simulink model "TST_Rail_CtlLoopParaMeUn"  (R2016b)
settings: Solver=FixedStepDiscrete  StartTime=0.0  StopTime=simTime  FixedStep=sampleTime  RelTol=1e-3
values from neighbouring files (symbols this model uses):
  testCase = 1    [initTST_Rail_CtlLoopParaMeUn_001.m]
libraries: simulink x11, UnitTest_Lib x9
settings Model: Creator=zhengjinyan  LastModifiedBy=zhengjinyan
settings DebuggingCC: SignalRangeChecking=error

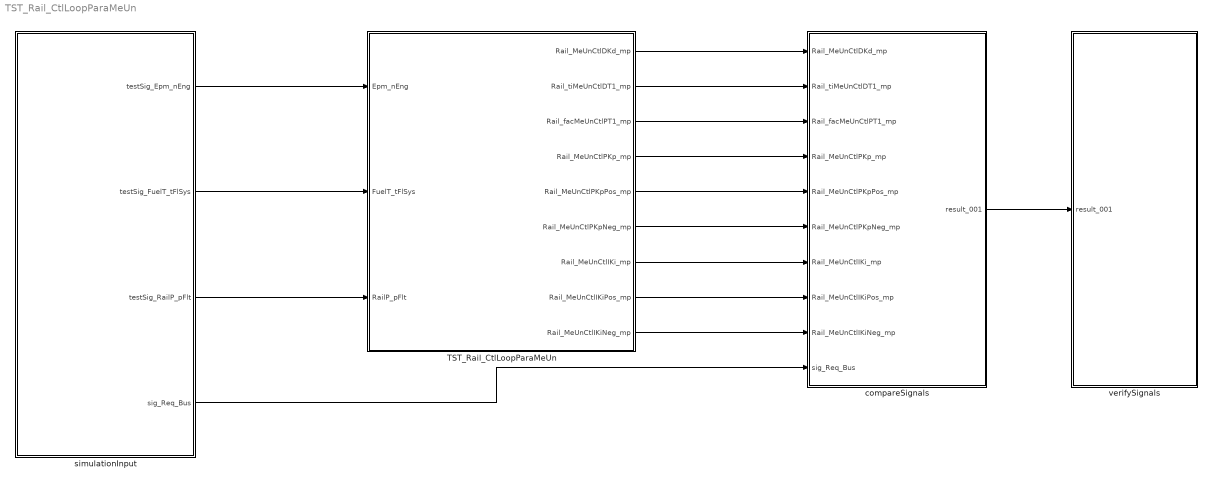
== system TST_Rail_CtlLoopParaMeUn ==
  TST_Rail_CtlLoopParaMeUn : Subsystem
  compareSignals : Subsystem
  simulationInput : Subsystem
  verifySignals : Subsystem
  wires:
  simulationInput/1(testSig_Epm_nEng) -> TST_Rail_CtlLoopParaMeUn/1(Epm_nEng)
  simulationInput/2(testSig_FuelT_tFlSys) -> TST_Rail_CtlLoopParaMeUn/2(FuelT_tFlSys)
  simulationInput/3(testSig_RailP_pFlt) -> TST_Rail_CtlLoopParaMeUn/3(RailP_pFlt)
  TST_Rail_CtlLoopParaMeUn/1(Rail_MeUnCtlDKd_mp) -> compareSignals/1(Rail_MeUnCtlDKd_mp)
  TST_Rail_CtlLoopParaMeUn/2(Rail_tiMeUnCtlDT1_mp) -> compareSignals/2(Rail_tiMeUnCtlDT1_mp)
  TST_Rail_CtlLoopParaMeUn/3(Rail_facMeUnCtlPT1_mp) -> compareSignals/3(Rail_facMeUnCtlPT1_mp)
  TST_Rail_CtlLoopParaMeUn/4(Rail_MeUnCtlPKp_mp) -> compareSignals/4(Rail_MeUnCtlPKp_mp)
  TST_Rail_CtlLoopParaMeUn/5(Rail_MeUnCtlPKpPos_mp) -> compareSignals/5(Rail_MeUnCtlPKpPos_mp)
  TST_Rail_CtlLoopParaMeUn/6(Rail_MeUnCtlPKpNeg_mp) -> compareSignals/6(Rail_MeUnCtlPKpNeg_mp)
  TST_Rail_CtlLoopParaMeUn/7(Rail_MeUnCtlIKi_mp) -> compareSignals/7(Rail_MeUnCtlIKi_mp)
  TST_Rail_CtlLoopParaMeUn/8(Rail_MeUnCtlIKiPos_mp) -> compareSignals/8(Rail_MeUnCtlIKiPos_mp)
  TST_Rail_CtlLoopParaMeUn/9(Rail_MeUnCtlIKiNeg_mp) -> compareSignals/9(Rail_MeUnCtlIKiNeg_mp)
  simulationInput/4(sig_Req_Bus) -> compareSignals/10(sig_Req_Bus)
  compareSignals/1(result_001) -> verifySignals/1(result_001)

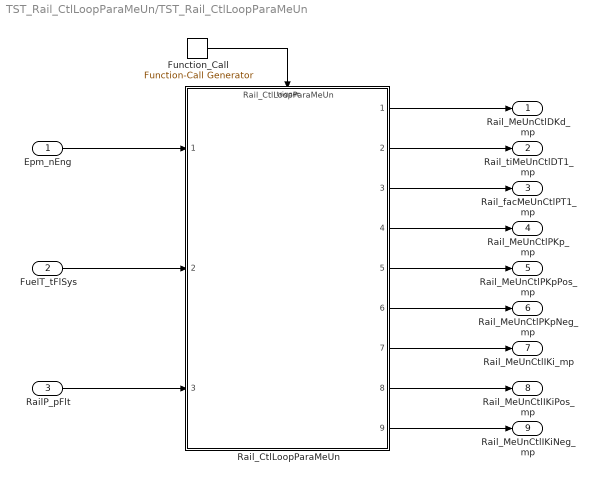
== system TST_Rail_CtlLoopParaMeUn/TST_Rail_CtlLoopParaMeUn ==
  Epm_nEng : Inport
  FuelT_tFlSys : Inport  Port=2
  RailP_pFlt : Inport  Port=3
  Function_Call : simulink/Ports & Subsystems/Function-Call Generator  sample_time=sampleTime  numberOfIterations=1
  Rail_CtlLoopParaMeUn : ModelReference  ModelNameDialog=Rail_CtlLoopParaMeUn  SimulationMode=Normal  ModelReferenceVersion=1.20  TriggerPortName=function  TriggerPortTriggerType=function-call  TriggerPortStatesWhenEnabling=held
  Rail_MeUnCtlDKd_mp : Outport
  Rail_tiMeUnCtlDT1_mp : Outport  Port=2
  Rail_facMeUnCtlPT1_mp : Outport  Port=3
  Rail_MeUnCtlPKp_mp : Outport  Port=4
  Rail_MeUnCtlPKpPos_mp : Outport  Port=5
  Rail_MeUnCtlPKpNeg_mp : Outport  Port=6
  Rail_MeUnCtlIKi_mp : Outport  Port=7
  Rail_MeUnCtlIKiPos_mp : Outport  Port=8
  Rail_MeUnCtlIKiNeg_mp : Outport  Port=9
  wires:
  Function_Call/1 -> Rail_CtlLoopParaMeUn/Trigger
  Epm_nEng/1 -> Rail_CtlLoopParaMeUn/1
  FuelT_tFlSys/1 -> Rail_CtlLoopParaMeUn/2
  RailP_pFlt/1 -> Rail_CtlLoopParaMeUn/3
  Rail_CtlLoopParaMeUn/1 -> Rail_MeUnCtlDKd_mp/1
  Rail_CtlLoopParaMeUn/2 -> Rail_tiMeUnCtlDT1_mp/1
  Rail_CtlLoopParaMeUn/3 -> Rail_facMeUnCtlPT1_mp/1
  Rail_CtlLoopParaMeUn/4 -> Rail_MeUnCtlPKp_mp/1
  Rail_CtlLoopParaMeUn/5 -> Rail_MeUnCtlPKpPos_mp/1
  Rail_CtlLoopParaMeUn/6 -> Rail_MeUnCtlPKpNeg_mp/1
  Rail_CtlLoopParaMeUn/7 -> Rail_MeUnCtlIKi_mp/1
  Rail_CtlLoopParaMeUn/8 -> Rail_MeUnCtlIKiPos_mp/1
  Rail_CtlLoopParaMeUn/9 -> Rail_MeUnCtlIKiNeg_mp/1

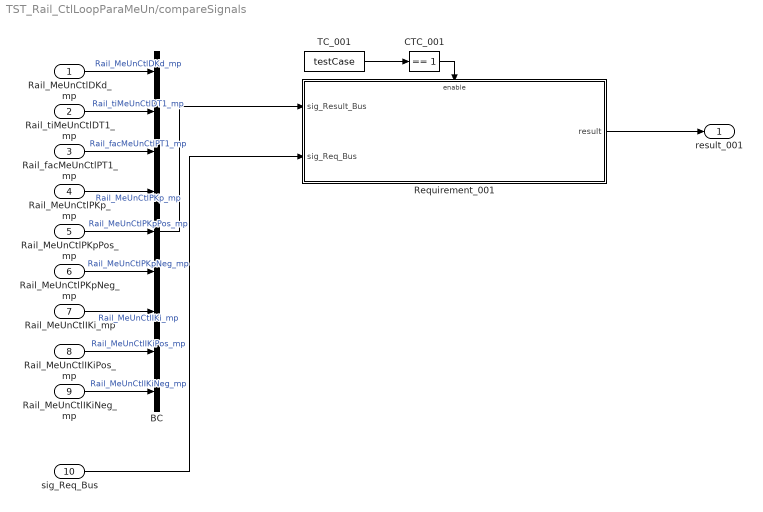
== system TST_Rail_CtlLoopParaMeUn/compareSignals ==
  Rail_MeUnCtlDKd_mp : Inport
  Rail_tiMeUnCtlDT1_mp : Inport  Port=2
  Rail_facMeUnCtlPT1_mp : Inport  Port=3
  Rail_MeUnCtlPKp_mp : Inport  Port=4
  Rail_MeUnCtlPKpPos_mp : Inport  Port=5
  Rail_MeUnCtlPKpNeg_mp : Inport  Port=6
  Rail_MeUnCtlIKi_mp : Inport  Port=7
  Rail_MeUnCtlIKiPos_mp : Inport  Port=8
  Rail_MeUnCtlIKiNeg_mp : Inport  Port=9
  sig_Req_Bus : Inport  Port=10
  BC : BusCreator  Inputs=9
  CTC_001 : simulink/Logic and Bit Operations/Compare To Constant  relop===  const=1  OutDataTypeStr=boolean
  Requirement_001 : Subsystem
  TC_001 : Constant  Value=testCase
  result_001 : Outport
  wires:
  Rail_MeUnCtlDKd_mp/1 -> BC/1  "Rail_MeUnCtlDKd_mp"
  Rail_tiMeUnCtlDT1_mp/1 -> BC/2  "Rail_tiMeUnCtlDT1_mp"
  Rail_facMeUnCtlPT1_mp/1 -> BC/3  "Rail_facMeUnCtlPT1_mp"
  Rail_MeUnCtlPKp_mp/1 -> BC/4  "Rail_MeUnCtlPKp_mp"
  Rail_MeUnCtlPKpPos_mp/1 -> BC/5  "Rail_MeUnCtlPKpPos_mp"
  Rail_MeUnCtlPKpNeg_mp/1 -> BC/6  "Rail_MeUnCtlPKpNeg_mp"
  Rail_MeUnCtlIKi_mp/1 -> BC/7  "Rail_MeUnCtlIKi_mp"
  Rail_MeUnCtlIKiPos_mp/1 -> BC/8  "Rail_MeUnCtlIKiPos_mp"
  Rail_MeUnCtlIKiNeg_mp/1 -> BC/9  "Rail_MeUnCtlIKiNeg_mp"
  TC_001/1 -> CTC_001/1
  CTC_001/1 -> Requirement_001/Enable
  sig_Req_Bus/1 -> Requirement_001/2(sig_Req_Bus)
  BC/1 -> Requirement_001/1(sig_Result_Bus)
  Requirement_001/1(result) -> result_001/1

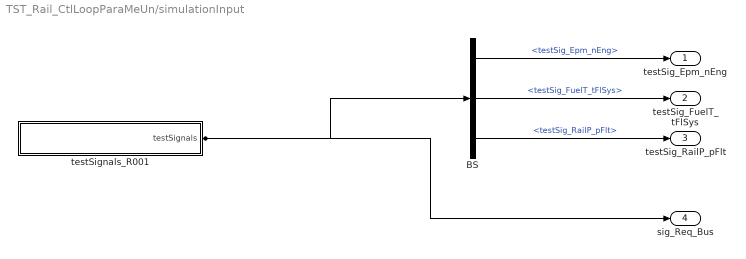
== system TST_Rail_CtlLoopParaMeUn/simulationInput ==
  BS : BusSelector  OutputSignals=testSig_Epm_nEng,testSig_FuelT_tFlSys,testSig_RailP_pFlt
  testSignals_R001 : Subsystem
  testSig_Epm_nEng : Outport
  testSig_FuelT_tFlSys : Outport  Port=2
  testSig_RailP_pFlt : Outport  Port=3
  sig_Req_Bus : Outport  Port=4
  wires:
  BS/1 -> testSig_Epm_nEng/1  "<testSig_Epm_nEng>"
  BS/2 -> testSig_FuelT_tFlSys/1  "<testSig_FuelT_tFlSys>"
  BS/3 -> testSig_RailP_pFlt/1  "<testSig_RailP_pFlt>"
  testSignals_R001/1(testSignals) -> BS/1, sig_Req_Bus/1

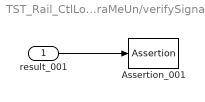
== system TST_Rail_CtlLoopParaMeUn/verifySignals ==
  result_001 : Inport
  Assertion_001 : Assertion  Enabled=off
  wires:
  result_001/1 -> Assertion_001/1

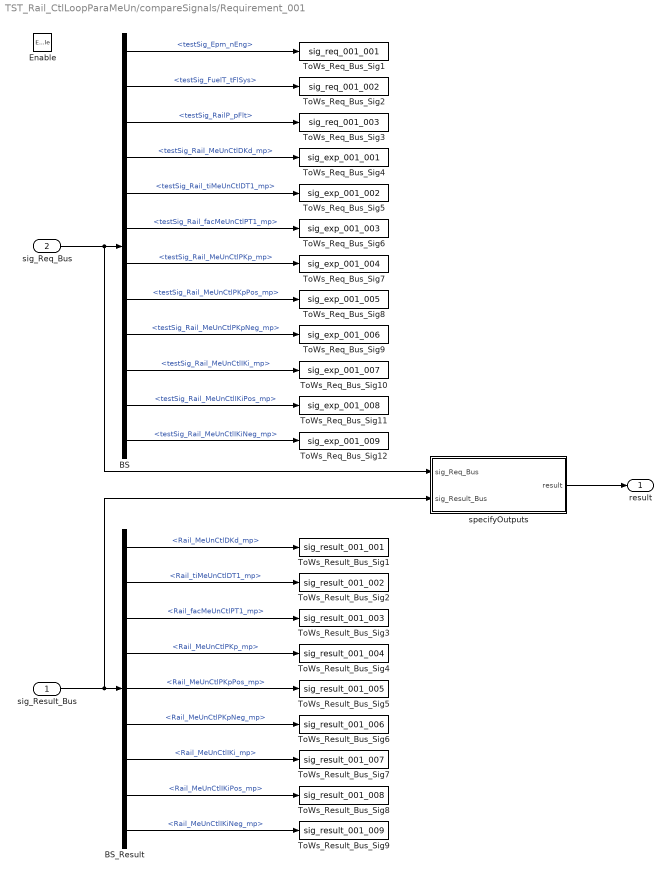
== system TST_Rail_CtlLoopParaMeUn/compareSignals/Requirement_001 ==
  sig_Result_Bus : Inport
  sig_Req_Bus : Inport  Port=2
  Enable : EnablePort
  BS : BusSelector  OutputSignals=testSig_Epm_nEng,testSig_FuelT_tFlSys,testSig_RailP_pFlt,testSig_Rail_MeUnCtlDKd_mp,testSig_Rail_tiMeUnCtlDT1_mp,testSig_Rail_facMeUnCtlPT1_mp,testSig_Rail_MeUnCtlPKp_mp,testSig_Rail_MeUnCtlPKpPos_mp,testSig_Rail_MeUnCtlPKpNeg_mp,testSig_Rail_MeUnCtlIKi_mp,testSig_Rail_MeUnCtlIKiPos_mp,testSig_Rail_MeUnCtlIKiNeg_mp
  BS_Result : BusSelector  OutputSignals=Rail_MeUnCtlDKd_mp,Rail_tiMeUnCtlDT1_mp,Rail_facMeUnCtlPT1_mp,Rail_MeUnCtlPKp_mp,Rail_MeUnCtlPKpPos_mp,Rail_MeUnCtlPKpNeg_mp,Rail_MeUnCtlIKi_mp,Rail_MeUnCtlIKiPos_mp,Rail_MeUnCtlIKiNeg_mp
  ToWs_Req_Bus_Sig1 : ToWorkspace  VariableName=sig_req_001_001  SaveFormat=Structure With Time
  ToWs_Req_Bus_Sig10 : ToWorkspace  VariableName=sig_exp_001_007  SaveFormat=Structure With Time
  ToWs_Req_Bus_Sig11 : ToWorkspace  VariableName=sig_exp_001_008  SaveFormat=Structure With Time
  ToWs_Req_Bus_Sig12 : ToWorkspace  VariableName=sig_exp_001_009  SaveFormat=Structure With Time
  ToWs_Req_Bus_Sig2 : ToWorkspace  VariableName=sig_req_001_002  SaveFormat=Structure With Time
  ToWs_Req_Bus_Sig3 : ToWorkspace  VariableName=sig_req_001_003  SaveFormat=Structure With Time
  ToWs_Req_Bus_Sig4 : ToWorkspace  VariableName=sig_exp_001_001  SaveFormat=Structure With Time
  ToWs_Req_Bus_Sig5 : ToWorkspace  VariableName=sig_exp_001_002  SaveFormat=Structure With Time
  ToWs_Req_Bus_Sig6 : ToWorkspace  VariableName=sig_exp_001_003  SaveFormat=Structure With Time
  ToWs_Req_Bus_Sig7 : ToWorkspace  VariableName=sig_exp_001_004  SaveFormat=Structure With Time
  ToWs_Req_Bus_Sig8 : ToWorkspace  VariableName=sig_exp_001_005  SaveFormat=Structure With Time
  ToWs_Req_Bus_Sig9 : ToWorkspace  VariableName=sig_exp_001_006  SaveFormat=Structure With Time
  ToWs_Result_Bus_Sig1 : ToWorkspace  VariableName=sig_result_001_001  SaveFormat=Structure With Time
  ToWs_Result_Bus_Sig2 : ToWorkspace  VariableName=sig_result_001_002  SaveFormat=Structure With Time
  ToWs_Result_Bus_Sig3 : ToWorkspace  VariableName=sig_result_001_003  SaveFormat=Structure With Time
  ToWs_Result_Bus_Sig4 : ToWorkspace  VariableName=sig_result_001_004  SaveFormat=Structure With Time
  ToWs_Result_Bus_Sig5 : ToWorkspace  VariableName=sig_result_001_005  SaveFormat=Structure With Time
  ToWs_Result_Bus_Sig6 : ToWorkspace  VariableName=sig_result_001_006  SaveFormat=Structure With Time
  ToWs_Result_Bus_Sig7 : ToWorkspace  VariableName=sig_result_001_007  SaveFormat=Structure With Time
  ToWs_Result_Bus_Sig8 : ToWorkspace  VariableName=sig_result_001_008  SaveFormat=Structure With Time
  ToWs_Result_Bus_Sig9 : ToWorkspace  VariableName=sig_result_001_009  SaveFormat=Structure With Time
  specifyOutputs : Subsystem
  result : Outport
  wires:
  sig_Req_Bus/1 -> BS/1, specifyOutputs/1(sig_Req_Bus)
  BS/1 -> ToWs_Req_Bus_Sig1/1  "<testSig_Epm_nEng>"
  BS/2 -> ToWs_Req_Bus_Sig2/1  "<testSig_FuelT_tFlSys>"
  BS/3 -> ToWs_Req_Bus_Sig3/1  "<testSig_RailP_pFlt>"
  BS/4 -> ToWs_Req_Bus_Sig4/1  "<testSig_Rail_MeUnCtlDKd_mp>"
  BS/5 -> ToWs_Req_Bus_Sig5/1  "<testSig_Rail_tiMeUnCtlDT1_mp>"
  BS/6 -> ToWs_Req_Bus_Sig6/1  "<testSig_Rail_facMeUnCtlPT1_mp>"
  BS/7 -> ToWs_Req_Bus_Sig7/1  "<testSig_Rail_MeUnCtlPKp_mp>"
  BS/8 -> ToWs_Req_Bus_Sig8/1  "<testSig_Rail_MeUnCtlPKpPos_mp>"
  BS/9 -> ToWs_Req_Bus_Sig9/1  "<testSig_Rail_MeUnCtlPKpNeg_mp>"
  BS/10 -> ToWs_Req_Bus_Sig10/1  "<testSig_Rail_MeUnCtlIKi_mp>"
  BS/11 -> ToWs_Req_Bus_Sig11/1  "<testSig_Rail_MeUnCtlIKiPos_mp>"
  BS/12 -> ToWs_Req_Bus_Sig12/1  "<testSig_Rail_MeUnCtlIKiNeg_mp>"
  sig_Result_Bus/1 -> BS_Result/1, specifyOutputs/2(sig_Result_Bus)
  BS_Result/1 -> ToWs_Result_Bus_Sig1/1  "<Rail_MeUnCtlDKd_mp>"
  BS_Result/2 -> ToWs_Result_Bus_Sig2/1  "<Rail_tiMeUnCtlDT1_mp>"
  BS_Result/3 -> ToWs_Result_Bus_Sig3/1  "<Rail_facMeUnCtlPT1_mp>"
  BS_Result/4 -> ToWs_Result_Bus_Sig4/1  "<Rail_MeUnCtlPKp_mp>"
  BS_Result/5 -> ToWs_Result_Bus_Sig5/1  "<Rail_MeUnCtlPKpPos_mp>"
  BS_Result/6 -> ToWs_Result_Bus_Sig6/1  "<Rail_MeUnCtlPKpNeg_mp>"
  BS_Result/7 -> ToWs_Result_Bus_Sig7/1  "<Rail_MeUnCtlIKi_mp>"
  BS_Result/8 -> ToWs_Result_Bus_Sig8/1  "<Rail_MeUnCtlIKiPos_mp>"
  BS_Result/9 -> ToWs_Result_Bus_Sig9/1  "<Rail_MeUnCtlIKiNeg_mp>"
  specifyOutputs/1(result) -> result/1

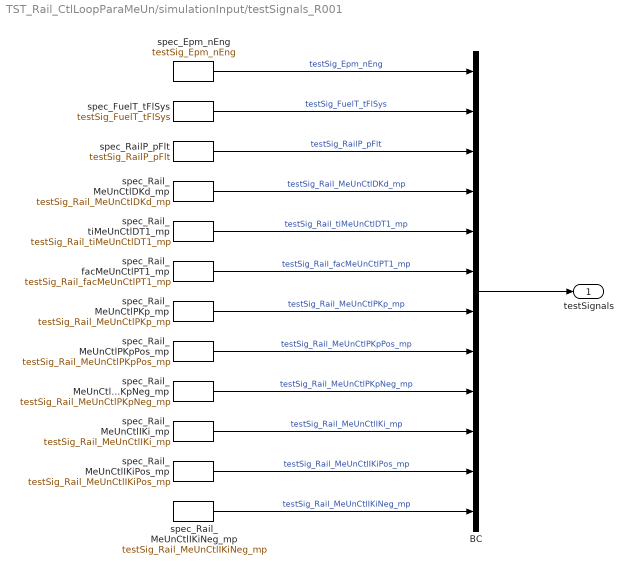
== system TST_Rail_CtlLoopParaMeUn/simulationInput/testSignals_R001 ==
  BC : BusCreator  Inputs=12
  spec_Epm_nEng : FromWorkspace  VariableName=testSig_Epm_nEng  Interpolate=off  OutputAfterFinalValue=Holding final value
  spec_FuelT_tFlSys : FromWorkspace  VariableName=testSig_FuelT_tFlSys  Interpolate=off  OutputAfterFinalValue=Holding final value
  spec_RailP_pFlt : FromWorkspace  VariableName=testSig_RailP_pFlt  Interpolate=off  OutputAfterFinalValue=Holding final value
  spec_Rail_MeUnCtlDKd_mp : FromWorkspace  VariableName=testSig_Rail_MeUnCtlDKd_mp  Interpolate=off  OutputAfterFinalValue=Holding final value
  spec_Rail_MeUnCtlIKiNeg_mp : FromWorkspace  VariableName=testSig_Rail_MeUnCtlIKiNeg_mp  Interpolate=off  OutputAfterFinalValue=Holding final value
  spec_Rail_MeUnCtlIKiPos_mp : FromWorkspace  VariableName=testSig_Rail_MeUnCtlIKiPos_mp  Interpolate=off  OutputAfterFinalValue=Holding final value
  spec_Rail_MeUnCtlIKi_mp : FromWorkspace  VariableName=testSig_Rail_MeUnCtlIKi_mp  Interpolate=off  OutputAfterFinalValue=Holding final value
  spec_Rail_MeUnCtlPKpNeg_mp : FromWorkspace  VariableName=testSig_Rail_MeUnCtlPKpNeg_mp  Interpolate=off  OutputAfterFinalValue=Holding final value
  spec_Rail_MeUnCtlPKpPos_mp : FromWorkspace  VariableName=testSig_Rail_MeUnCtlPKpPos_mp  Interpolate=off  OutputAfterFinalValue=Holding final value
  spec_Rail_MeUnCtlPKp_mp : FromWorkspace  VariableName=testSig_Rail_MeUnCtlPKp_mp  Interpolate=off  OutputAfterFinalValue=Holding final value
  spec_Rail_facMeUnCtlPT1_mp : FromWorkspace  VariableName=testSig_Rail_facMeUnCtlPT1_mp  Interpolate=off  OutputAfterFinalValue=Holding final value
  spec_Rail_tiMeUnCtlDT1_mp : FromWorkspace  VariableName=testSig_Rail_tiMeUnCtlDT1_mp  Interpolate=off  OutputAfterFinalValue=Holding final value
  testSignals : Outport
  wires:
  BC/1 -> testSignals/1
  spec_Epm_nEng/1 -> BC/1  "testSig_Epm_nEng"
  spec_FuelT_tFlSys/1 -> BC/2  "testSig_FuelT_tFlSys"
  spec_RailP_pFlt/1 -> BC/3  "testSig_RailP_pFlt"
  spec_Rail_MeUnCtlDKd_mp/1 -> BC/4  "testSig_Rail_MeUnCtlDKd_mp"
  spec_Rail_tiMeUnCtlDT1_mp/1 -> BC/5  "testSig_Rail_tiMeUnCtlDT1_mp"
  spec_Rail_facMeUnCtlPT1_mp/1 -> BC/6  "testSig_Rail_facMeUnCtlPT1_mp"
  spec_Rail_MeUnCtlPKp_mp/1 -> BC/7  "testSig_Rail_MeUnCtlPKp_mp"
  spec_Rail_MeUnCtlPKpPos_mp/1 -> BC/8  "testSig_Rail_MeUnCtlPKpPos_mp"
  spec_Rail_MeUnCtlPKpNeg_mp/1 -> BC/9  "testSig_Rail_MeUnCtlPKpNeg_mp"
  spec_Rail_MeUnCtlIKi_mp/1 -> BC/10  "testSig_Rail_MeUnCtlIKi_mp"
  spec_Rail_MeUnCtlIKiPos_mp/1 -> BC/11  "testSig_Rail_MeUnCtlIKiPos_mp"
  spec_Rail_MeUnCtlIKiNeg_mp/1 -> BC/12  "testSig_Rail_MeUnCtlIKiNeg_mp"

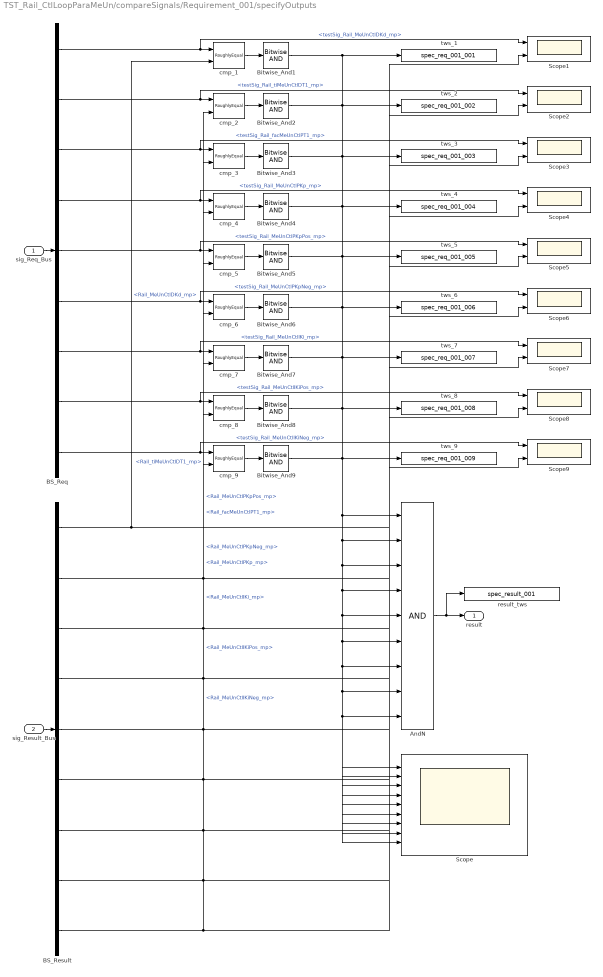
== system TST_Rail_CtlLoopParaMeUn/compareSignals/Requirement_001/specifyOutputs ==
  sig_Req_Bus : Inport
  sig_Result_Bus : Inport  Port=2
  AndN : Logic  Inputs=9
  BS_Req : BusSelector  OutputSignals=testSig_Rail_MeUnCtlDKd_mp,testSig_Rail_tiMeUnCtlDT1_mp,testSig_Rail_facMeUnCtlPT1_mp,testSig_Rail_MeUnCtlPKp_mp,testSig_Rail_MeUnCtlPKpPos_mp,testSig_Rail_MeUnCtlPKpNeg_mp,testSig_Rail_MeUnCtlIKi_mp,testSig_Rail_MeUnCtlIKiPos_mp,testSig_Rail_MeUnCtlIKiNeg_mp
  BS_Result : BusSelector  OutputSignals=Rail_MeUnCtlDKd_mp,Rail_tiMeUnCtlDT1_mp,Rail_facMeUnCtlPT1_mp,Rail_MeUnCtlPKp_mp,Rail_MeUnCtlPKpPos_mp,Rail_MeUnCtlPKpNeg_mp,Rail_MeUnCtlIKi_mp,Rail_MeUnCtlIKiPos_mp,Rail_MeUnCtlIKiNeg_mp
  Bitwise_And{1..9} (9 alike) : simulink/Logic and Bit Operations/Bitwise Operator  logicop=AND  UseBitMask=off  BitMask=bin2dec('11011001')  BitMaskRealWorld=Stored Integer
  Scope : Scope  NumInputPorts=9
  Scope{1..9} (9 alike) : Scope  NumInputPorts=2
  cmp_1 : UnitTest_Lib/RoughlyEqual  slope=0.1
  cmp_{2..9} (8 alike) : UnitTest_Lib/RoughlyEqual  slope=1
  result_tws : ToWorkspace  VariableName=spec_result_001
  tws_1 : ToWorkspace  VariableName=spec_req_001_001
  tws_2 : ToWorkspace  VariableName=spec_req_001_002
  tws_3 : ToWorkspace  VariableName=spec_req_001_003
  tws_4 : ToWorkspace  VariableName=spec_req_001_004
  tws_5 : ToWorkspace  VariableName=spec_req_001_005
  tws_6 : ToWorkspace  VariableName=spec_req_001_006
  tws_7 : ToWorkspace  VariableName=spec_req_001_007
  tws_8 : ToWorkspace  VariableName=spec_req_001_008
  tws_9 : ToWorkspace  VariableName=spec_req_001_009
  result : Outport
  wires:
  sig_Req_Bus/1 -> BS_Req/1
  sig_Result_Bus/1 -> BS_Result/1
  AndN/1 -> result/1, result_tws/1
  BS_Req/1 -> cmp_1/1, Scope1/1  "<testSig_Rail_MeUnCtlDKd_mp>"
  BS_Result/1 -> cmp_1/2, Scope1/2  "<Rail_MeUnCtlDKd_mp>"
  cmp_1/1 -> Bitwise_And1/1
  Bitwise_And1/1 -> AndN/1, Scope/1, tws_1/1
  BS_Req/2 -> cmp_2/1, Scope2/1  "<testSig_Rail_tiMeUnCtlDT1_mp>"
  BS_Result/2 -> cmp_2/2, Scope2/2  "<Rail_tiMeUnCtlDT1_mp>"
  cmp_2/1 -> Bitwise_And2/1
  Bitwise_And2/1 -> AndN/2, Scope/2, tws_2/1
  BS_Req/3 -> cmp_3/1, Scope3/1  "<testSig_Rail_facMeUnCtlPT1_mp>"
  BS_Result/3 -> cmp_3/2, Scope3/2  "<Rail_facMeUnCtlPT1_mp>"
  cmp_3/1 -> Bitwise_And3/1
  Bitwise_And3/1 -> AndN/3, Scope/3, tws_3/1
  BS_Req/4 -> cmp_4/1, Scope4/1  "<testSig_Rail_MeUnCtlPKp_mp>"
  BS_Result/4 -> cmp_4/2, Scope4/2  "<Rail_MeUnCtlPKp_mp>"
  cmp_4/1 -> Bitwise_And4/1
  Bitwise_And4/1 -> AndN/4, Scope/4, tws_4/1
  BS_Req/5 -> cmp_5/1, Scope5/1  "<testSig_Rail_MeUnCtlPKpPos_mp>"
  BS_Result/5 -> cmp_5/2, Scope5/2  "<Rail_MeUnCtlPKpPos_mp>"
  cmp_5/1 -> Bitwise_And5/1
  Bitwise_And5/1 -> AndN/5, Scope/5, tws_5/1
  BS_Req/6 -> cmp_6/1, Scope6/1  "<testSig_Rail_MeUnCtlPKpNeg_mp>"
  BS_Result/6 -> cmp_6/2, Scope6/2  "<Rail_MeUnCtlPKpNeg_mp>"
  cmp_6/1 -> Bitwise_And6/1
  Bitwise_And6/1 -> AndN/6, Scope/6, tws_6/1
  BS_Req/7 -> cmp_7/1, Scope7/1  "<testSig_Rail_MeUnCtlIKi_mp>"
  BS_Result/7 -> cmp_7/2, Scope7/2  "<Rail_MeUnCtlIKi_mp>"
  cmp_7/1 -> Bitwise_And7/1
  Bitwise_And7/1 -> AndN/7, Scope/7, tws_7/1
  BS_Req/8 -> cmp_8/1, Scope8/1  "<testSig_Rail_MeUnCtlIKiPos_mp>"
  BS_Result/8 -> cmp_8/2, Scope8/2  "<Rail_MeUnCtlIKiPos_mp>"
  cmp_8/1 -> Bitwise_And8/1
  Bitwise_And8/1 -> AndN/8, Scope/8, tws_8/1
  BS_Req/9 -> cmp_9/1, Scope9/1  "<testSig_Rail_MeUnCtlIKiNeg_mp>"
  BS_Result/9 -> cmp_9/2, Scope9/2  "<Rail_MeUnCtlIKiNeg_mp>"
  cmp_9/1 -> Bitwise_And9/1
  Bitwise_And9/1 -> AndN/9, Scope/9, tws_9/1
